simulink model "SA_50"  (R2021a)
settings: Solver=VariableStepAuto  StartTime=0.0  StopTime=simTime  RelTol=1e-3
model workspace (MAT data in the model file):
  SoC_0 = Simulink.Parameter
  SoC_0.DataType = 'auto'
  SoC_0.Dimensions = [0 0]
undefined symbols (not defined in the file or in its folder): Ion, Lithium, sigbuilder_block, slow_linearMPC
libraries: spsCurrentMeasurementLib x3, spsSeriesRLCBranchLib x2, spsDiodeLib x2, spspowerguiLib x1, spsBatteryLib x1, spsControlledCurrentSourceLib x1, spsFirstOrderFilterLib x1, spsFuelCellStackLib x1, spsMosfetLib x1, pid_lib x1, spsPWMGeneratorDCDCLib x1
settings Model: SimulationMode=accelerator  OrderedModelArguments=off  Creator=g  LastModifiedBy=leonardopalacios
settings SolverCC: ZeroCrossControl=DisableAll  ZeroCrossAlgorithm=Adaptive  AlgebraicLoopSolver=TrustRegion
settings DataIOCC: ReturnWorkspaceOutputs=off
settings DebuggingCC: SFMachineParentedDataDiag=warning  ArithmeticOperatorsInVariantConditions=warning
settings SFSimCC: SimUseLocalCustomCode=off  CustomCodeUndefinedFunction=UseInterfaceOnly
settings RTWCC: RTWUseLocalCustomCode=off
settings CodeAppCC: StateflowObjectComments=on
settings SimscapeCC: SimscapeNormalizeSystem=off

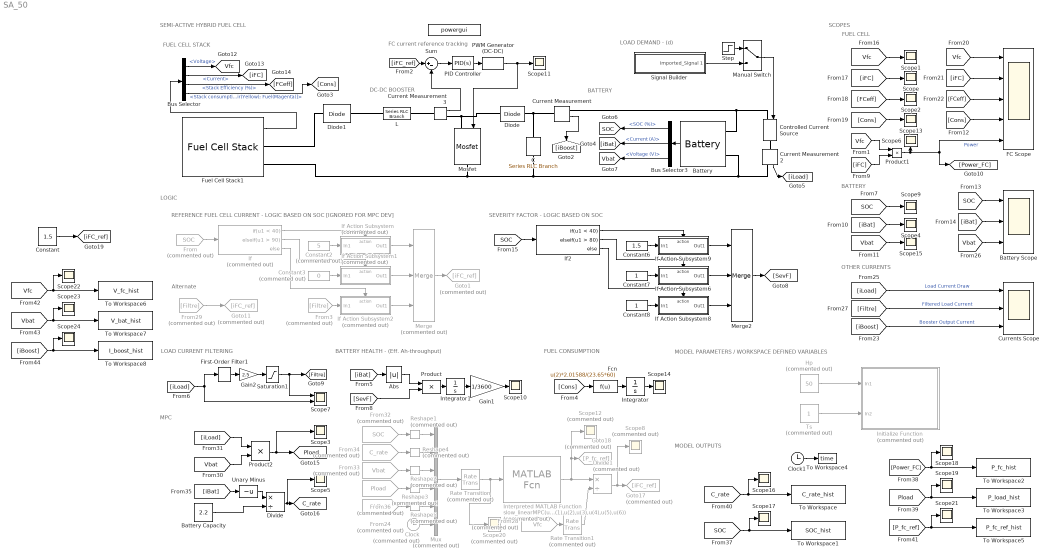
== system SA_50 ==
  note: MPC
  note: Alternate
  note: MODEL PARAMETERS / WORKSPACE DEFINED VARIABLES
  note: SCOPES
  note: SEMI-ACTIVE HYBRID FUEL CELL
  note: LOAD CURRENT FILTERING
  note: LOGIC
  note: LOAD DEMAND - (d)
  note: BATTERY
  note: REFERENCE FUEL CELL CURRENT - LOGIC BASED ON SOC [IGNORED FOR MPC DEV]
  note: FC current reference tracking
  note: DC-DC BOOSTER
  note: BATTERY
  note: FUEL CELL
  note: OTHER CURRENTS
  note: SEVERITY FACTOR - LOGIC BASED ON SOC
  note: FUEL CELL STACK
  note: BATTERY HEALTH - (Eff. Ah-throughput)
  note: FUEL CONSUMPTION
  note: MODEL OUTPUTS
  " " : spspowerguiLib/powergui  Priority=1  SimulationMode=Continuous  SampleTime=50e-6  frequency=60  Iterations=50  frequencyindice=0  Pbase=100e6  ErrMax=1e-4  UnitsV=kV  UnitsW=MW  buscounter=0  FunctionMessages=off  echomessages=off  EnableUseOfTLC=off  CurrentSourceSwitches=off  DisableSnubberDevices=off  DisableRonSwitches=off  DisableVfSwitches=off  DisplayEquations=off  AutomaticDiscreteSolvers=off  SolverType=Tustin/Backward Euler (TBE)  Interpol=off  ExternalGateDelay=off  methode=off  Ts=10  x0status=blocks  SPID=off  SwTol=0  HookPort=off  NonlinearTolerance=1e-4  nMaxIteration=100  ContinueOnMaxIteration=off  RestoreLinks=warning  ResistiveCurrentMeasurement=off  Frange=[0:2:500]  Ylog=off  Xlog=on  ShowGrid=off  save=off  variable=ZData  structure=0  ZoomFFT=off  StartTime=0.0  cycles=1  DisplayStyle=1  fundamental=60  FreqAxis=off  MaxFrequency=1000  frequencyindicesteady=1  RmsSteady=1  display=off
  Abs : Abs
  Battery : spsBatteryLib/Battery  BatType=Lithium-Ion  ShowTempParam=off  ThermalPreset=no  ShowAgeParam=off  NomV=40  NomQ=2.2  SOC=50  Batt_Tr=30  PresetModel=on  MaxQ=2.2  MinV=30  FullV=46.5595  Dis_rate=0.95652  R=0.18182  Normal_OP=1.9896  expZone="[43.2154     0.108087]"  current=[6.5 13 32.5]  Units=Time  Tci=20  NomT=25  T2=0  MaxQ2=2.208  FullV2=3.45  Normal_OP2=2.8  expZone2="[3.22        0.23]"  Rca=0.6  ti=1000  Dp=0  Neq0=0  Tsim=1e6  Ta1=25  Qeol=5.4*0.9  Reol=0.013333*1.2  Char_age=[2.3478, 3]  Dis_age=[2.3478, 10]  N1=1500  N2=10500  N3=1000  N4=1400  Ta2=45  N5=950
  Battery Capacity : Constant  Value=2.2
  "Battery Scope " : Scope  NumInputPorts=3
  Bus Selector : BusSelector  OutputSignals=Voltage,Current,Stack Efficiency (%),Stack consumption (Standard lpm) [Air(Yellow); Fuel(Magenta)]
  Bus Selector3 : BusSelector  OutputSignals=SOC (%),Current (A),Voltage (V)
  C : spsSeriesRLCBranchLib/Series RLC Branch  LConnTagsString=__new0  RConnTagsString=__new0  BranchType=C  Resistance=1  Inductance=100e-6  SetiL0=off  InitialCurrent=0  Capacitance=1000e-6  Setx0=off  InitialVoltage=0  Measurements=None
  Clock : Clock  Commented=on
  Clock1 : Clock
  Constant : Constant  Value=1.5
  Constant2 : Constant  Commented=on  Value=5
  Constant3 : Constant  Commented=on  Value=0
  Constant6 : Constant  Value=1.5
  Constant7 : Constant
  Constant8 : Constant
  Controlled Current Source : spsControlledCurrentSourceLib/Controlled Current Source  Initialize=off  Source_Type=DC  Amplitude=0  Phase=0  Frequency=0  Measurements=Current
  Current Measurement : spsCurrentMeasurementLib/Current Measurement  PhasorSimulation=off  OutputType=Complex  PSBequivalent=0
  Current Measurement2 : spsCurrentMeasurementLib/Current Measurement  PhasorSimulation=off  OutputType=Complex  PSBequivalent=0
  Current Measurement3 : spsCurrentMeasurementLib/Current Measurement  PhasorSimulation=off  OutputType=Complex  PSBequivalent=0
  "Currents Scope " : Scope  NumInputPorts=3
  Diode : spsDiodeLib/Diode  Ron=0.001  Lon=0  Vf=0.8  IC=0  UseSnubber=off  Rs=500  Cs=250e-9  Measurements=off
  Diode1 : spsDiodeLib/Diode  Ron=0.001  Lon=0  Vf=0.8  IC=0  UseSnubber=off  Rs=500  Cs=250e-9  Measurements=off
  Divide : Product  Inputs=*/
  Divide1 : Product  Commented=on  Inputs=*/
  FC Scope : Scope  NumInputPorts=5
  Fcn : Fcn  Expr=u(2)*2.01588/(23.65*60)
  First-Order Filter1 : spsFirstOrderFilterLib/First-Order Filter  FilterType=Lowpass  Tc=5  Ts=0  Initialize=on  Vac_Init=[0, 0, 60]  Vdc_Init=1.1  PlotResponse=off  FreqRange="[0,  200,  1]"
  From : From  Commented=on  GotoTag=SOC
  From24 : From  Commented=on  GotoTag=Vfc  TagVisibility=global
  From28 : From  Commented=on  GotoTag=Vfc  TagVisibility=global
  From29 : From  Commented=on  GotoTag=Filtre
  From3 : From  Commented=on  GotoTag=Filtre
  From32 : From  Commented=on  GotoTag=SOC  TagVisibility=global
  From33 : From  Commented=on  GotoTag=Vbat  TagVisibility=global
  From34 : From  Commented=on  GotoTag=C_rate  TagVisibility=global
  From36 : From  Commented=on  GotoTag=Pload  TagVisibility=global
  Fuel Cell Stack1 : spsFuelCellStackLib/Fuel Cell Stack  PresetModel=No (User-Defined)  FcType=0  Detailed=Detailed  Eoc="[18  15]"  NomVI="[4        12.5]"  EndVI="[5   12]"  Nc=20  n=46  TOp=25  AirFr=20  SuppPress="[0.35           0.3]"  Comp="[99.95           21            1]"  SignX=off  SignY=off  FlowRateH2=off  FlowRateAir=off  SystemTemp=off  SystemPH2=off  SystemPAir=off  FCDyn=off  FC_tau=1  Peak_O2=80  V_Under=10
      settings: SourceProductBaseCode=PS
  Gain1 : Gain  Gain=1/3600
  Gain2 : Gain  Gain=2.5
  Goto1 : Goto  Commented=on  GotoTag=iFC_ref
  Goto11 : Goto  Commented=on  GotoTag=iFC_ref
  Goto17 : Goto  Commented=on  GotoTag=iFC_ref
  Goto18 : Goto  Commented=on  GotoTag=P_fc_ref
  Hp : Constant  Commented=on  Value=50
  If : If  Commented=on  IfExpression=u1 < 40  ElseIfExpressions=u1 > 90
  If Action Subsystem : Subsystem  Commented=on  TreatAsAtomicUnit=on
  If Action Subsystem1 : Subsystem  Commented=on  TreatAsAtomicUnit=on
  If Action Subsystem2 : Subsystem  Commented=on  TreatAsAtomicUnit=on
  If Action Subsystem6 : Subsystem  TreatAsAtomicUnit=on
  If Action Subsystem8 : Subsystem  TreatAsAtomicUnit=on
  If Action Subsystem9 : Subsystem  TreatAsAtomicUnit=on
  If2 : If  IfExpression=u1 < 40  ElseIfExpressions=u1 > 80
  Initialize Function : Subsystem  Commented=on  TreatAsAtomicUnit=on
  Integrator : Integrator
  Integrator1 : Integrator
  Interpreted MATLAB Function : MATLABFcn  Commented=on  MATLABFcn=slow_linearMPC(u(1),u(2),u(3),u(4),u(5),u(6))
  L : spsSeriesRLCBranchLib/Series RLC Branch  LConnTagsString=__new0  RConnTagsString=__new0  BranchType=L  Resistance=1  Inductance=100e-3  SetiL0=off  InitialCurrent=0  Capacitance=1e-6  Setx0=off  InitialVoltage=0  Measurements=None
  Manual Switch : ManualSwitch
  Merge : Merge  Commented=on  Inputs=3
  Merge2 : Merge  Inputs=3
  Mosfet : spsMosfetLib/Mosfet  Ron=0.1  Lon=0  Rd=0.01  Vfd=0  IC=0  Rs=1e5  Cs=inf  Measurements=off
  Mux : Mux  Commented=on  Inputs=6
  PID Controller : pid_lib/PID Controller  Controller=PID  Form=Parallel  TimeDomain=Continuous-time  UseExternalTs=off  SampleTime=-1  IntegratorMethod=Forward Euler  FilterMethod=Forward Euler  ControllerParametersSource=internal  P=1  I=2  D=0  UseFilter=on  N=100  TunerSelectOption=Transfer Function Based (PID Tuner App)  InitialConditionSource=internal  InitialConditionForIntegrator=0  InitialConditionForFilter=0  DifferentiatorICPrevScaledInput=0  ExternalReset=none  TrackingMode=off  Kt=1  LimitOutput=off  SatLimitsSource=internal  UpperSaturationLimit=inf  LowerSaturationLimit=-inf  LinearizeAsGain=on  AntiWindupMode=none  Kb=1  POutMin=[]  POutMax=[]  IOutMin=[]  IOutMax=[]  DOutMin=[]  DOutMax=[]  NOutMin=[]  NOutMax=[]  SumOutMin=[]  SumOutMax=[]  SaturationOutMin=[]  SaturationOutMax=[]  PParamMin=[]  PParamMax=[]  IParamMin=[]  IParamMax=[]  DParamMin=[]  DParamMax=[]  NParamMin=[]  NParamMax=[]  KbParamMin=[]  KbParamMax=[]  KtParamMin=[]  KtParamMax=[]  KbOutMin=[]  KbOutMax=[]  KtOutMin=[]  KtOutMax=[]  IntegratorOutMin=[]  IntegratorOutMax=[]  FilterOutMin=[]  FilterOutMax=[]  SumI1OutMin=[]  SumI1OutMax=[]  SumI2OutMin=[]  SumI2OutMax=[]  SumI3OutMin=[]  SumI3OutMax=[]  SumI4OutMin=[]  SumI4OutMax=[]  SumDOutMin=[]  SumDOutMax=[]  DifferentiatorOutMin=[]  DifferentiatorOutMax=[]  FilterDiffOutCoefMin=[]  FilterDiffOutCoefMax=[]  ReciprocalOutMin=[]  ReciprocalOutMax=[]  SumDenOutMin=[]  SumDenOutMax=[]  SumNumOutMin=[]  SumNumOutMax=[]  DivideOutMin=[]  DivideOutMax=[]  UdiffTsProdOutMin=[]  UdiffTsProdOutMax=[]  NTsProdOutMin=[]  NTsProdOutMax=[]  UintegralTsProdOutMin=[]  UintegralTsProdOutMax=[]  UngainTsProdOutMin=[]  UngainTsProdOutMax=[]  IntegratorContinuousStateAttributes=''  IntegratorStateMustResolveToSignalObject=off  IntegratorRTWStateStorageClass=Auto  FilterContinuousStateAttributes=''  FilterStateMustResolveToSignalObject=off  FilterRTWStateStorageClass=Auto  ParallelPVariant=InternalParameters  IdealPVariant=Disabled  IVariant=InternalParameters  DVariant=InternalParameters  IntegratorVariant=Continuous  SatVariant=Disabled  AWVariant=Passthrough  PCopyVariant=Disabled  TRVariant=Disabled  FdbkBlocksVariant=Forward  IdealPFdbkVariant=Disabled  SatFdbkVariant=Disabled  DerivativeFilterVariant=ContFilter  NVariant=InternalParameters  NCopyVariant=Disabled  FilterICVariant=InternalICsFilter  IntegratorICVariant=InternalICs  ExternalResetVariant=Disabled  TRSumVariant=Passthrough  SumFdbkVariant=Disabled  SumVariant=Sum_PID  TsampFilterVariant=InternalTs  TsampNgainVariant=Passthrough  TsampIntegralVariant=Passthrough  ExternalSaturationOutDataTypeStr=Inherit: Same as second input
  PWM Generator (DC-DC) : spsPWMGeneratorDCDCLib/PWM Generator (DC-DC)  Fsw=1000  Ts=0
  Product : Product
  Product1 : Product
  Product2 : Product
  Rate Transition : RateTransition  Commented=on  OutPortSampleTime=Ts
  Rate Transition1 : RateTransition  Commented=on  OutPortSampleTime=Ts
  Reshape{1..5} (5 alike) : Reshape  Commented=on  OutputDimensionality=Customize  OutputDimensions=1
  Saturation1 : Saturate  UpperLimit=5  LowerLimit=0
  Scope{,1..6,9..11,13..19,21..24} (21 alike) : Scope
  Scope12 : Scope  Commented=on
  Scope20 : Scope  Commented=on
  Scope7 : Scope  NumInputPorts=2
  Scope8 : Scope  Commented=on
  Signal Builder : Subsystem  Tag=STV Subsys  LoadFcn=sigbuilder_block('load');  StartFcn=sigbuilder_block('start');  StopFcn=sigbuilder_block('stop');  ClipboardFcn=sigbuilder_block('clipboard');  mask(Sigbuilder block){tuvar=[0:10]}
      mask help: Simulink:masks:SigbuilderBlock_MD
      mask init:
      | if ~strcmp(get_param(bdroot(gcbh),'SimulationStatus'),'stopped') tuvar = sigbuilder_block('maskInit'); end
      settings: CopyFcn=sigbuilder_block('copy');  DeleteFcn=sigbuilder_block('delete');  ModelCloseFcn=sigbuilder_block('modelClose');  PreSaveFcn=sigbuilder_block('preSave');  PauseFcn=sigbuilder_block('pause');  ContinueFcn=sigbuilder_block('continue');  NameChangeFcn=sigbuilder_block('namechange');  OpenFcn=sigbuilder_block('open',[214 20 1706 550 ]);  CloseFcn=sigbuilder_block('close');
      mask Display: plot(0, 0, 100, 100,[2, 2, 32, 32, 2], [68, 8, 8, 68, 68],[32, 2], [38, 38], [32, 19, 2],[53, 60, 44], [32, 17, 17, 2],[16, 16, 31, 31]);txt = getActiveGroup(gcbh);text(2, 100, txt,'verticalAlignment', 'top');
  Step : Step  Time=0  After=0.6  SampleTime=0
  Sum : Sum  Inputs=|+-
  To Workspace : ToWorkspace  VariableName=C_rate_hist  SaveFormat=Timeseries  SampleTime=-1
  To Workspace1 : ToWorkspace  VariableName=SOC_hist  SaveFormat=Timeseries  SampleTime=-1
  To Workspace2 : ToWorkspace  VariableName=P_fc_hist  SaveFormat=Timeseries  SampleTime=-1
  To Workspace3 : ToWorkspace  VariableName=P_load_hist  SaveFormat=Timeseries  SampleTime=-1
  To Workspace4 : ToWorkspace  VariableName=time  SaveFormat=Timeseries  SampleTime=-1
  To Workspace5 : ToWorkspace  VariableName=P_fc_ref_hist  SaveFormat=Timeseries  SampleTime=-1
  To Workspace6 : ToWorkspace  VariableName=V_fc_hist  SaveFormat=Timeseries  SampleTime=-1
  To Workspace7 : ToWorkspace  VariableName=V_bat_hist  SaveFormat=Timeseries  SampleTime=-1
  To Workspace8 : ToWorkspace  VariableName=I_boost_hist  SaveFormat=Timeseries  SampleTime=-1
  Ts : Constant  Commented=on
  Unary Minus : UnaryMinus
  tag scope: C_rate=global, Pload=global, SOC=global, Vbat=global, Vfc=global
  wires:
  Fuel Cell Stack1/1 -> Bus Selector/1
  [iFC_ref] -> Sum/1
  PWM Generator (DC-DC)/1 -> Mosfet/1, Scope11/1
  Current Measurement3/1 -> Sum/2
  From/1 -> If/1
  If/1 -> If Action Subsystem/Action
  If/2 -> If Action Subsystem1/Action
  If/3 -> If Action Subsystem2/Action
  Constant2/1 -> If Action Subsystem/1(In1)
  Constant3/1 -> If Action Subsystem1/1(In1)
  From3/1 -> If Action Subsystem2/1(In1)
  If Action Subsystem/1(Out1) -> Merge/1
  If Action Subsystem1/1(Out1) -> Merge/2
  If Action Subsystem2/1(Out1) -> Merge/3
  Merge/1 -> Goto1/1
  [Cons] -> Fcn/1
  Fcn/1 -> Integrator/1
  Integrator/1 -> Scope14/1
  [iBat] -> Abs/1
  Abs/1 -> Product/1
  [SevF] -> Product/2
  Product/1 -> Integrator1/1
  Bus Selector/4 -> [Cons]  "<Stack consumption (Standard lpm) [Air(Yellow); Fuel(Magenta)]>"
  Bus Selector/1 -> [Vfc]  "<Voltage>"
  Bus Selector/2 -> [iFC]  "<Current>"
  Bus Selector/3 -> [FCeff]  "<Stack Efficiency (%)>"
  [SOC] -> Scope9/1
  [iBat] -> Scope4/1
  [Vbat] -> Scope15/1
  [Vfc] -> Scope1/1
  [iFC] -> Scope/1
  [FCeff] -> Scope2/1
  [Cons] -> Scope13/1
  [Vfc] -> FC Scope/1
  [iFC] -> FC Scope/2
  [FCeff] -> FC Scope/3
  [Cons] -> FC Scope/4
  [SOC] -> "Battery Scope "/1
  [Vbat] -> "Battery Scope "/3
  Sum/1 -> PID Controller/1
  PID Controller/1 -> PWM Generator (DC-DC)/1
  Integrator1/1 -> Gain1/1
  Gain1/1 -> Scope10/1
  [Vfc] -> Product1/1
  [iFC] -> Product1/2
  [iBat] -> "Battery Scope "/2
  Product1/1 -> FC Scope/5, [Power_FC], Scope6/1  "Power"
  If2/3 -> If Action Subsystem8/Action
  If2/1 -> If Action Subsystem9/Action
  Constant6/1 -> If Action Subsystem9/1(In1)
  Merge2/1 -> [SevF]
  Constant8/1 -> If Action Subsystem8/1(In1)
  If Action Subsystem9/1(Out1) -> Merge2/1
  Constant7/1 -> If Action Subsystem6/1(In1)
  If Action Subsystem6/1(Out1) -> Merge2/2
  [SOC] -> If2/1
  If2/2 -> If Action Subsystem6/Action
  If Action Subsystem8/1(Out1) -> Merge2/3
  Gain2/1 -> Saturation1/1
  Saturation1/1 -> [Filtre], Scope7/1
  First-Order Filter1/1 -> Gain2/1
  [iLoad] -> Scope7/2, First-Order Filter1/1
  Current Measurement2/1 -> [iLoad]
  Current Measurement/1 -> [iBoost]
  [iLoad] -> "Currents Scope "/1  "Load Current Draw"
  [Filtre] -> "Currents Scope "/2  "Filtered Load Current"
  [iBoost] -> "Currents Scope "/3  "Booster Output Current"
  From29/1 -> Goto11/1
  Step/1 -> Manual Switch/1
  Signal Builder/1(Imported_Signal 1) -> Manual Switch/2
  Manual Switch/1 -> Controlled Current Source/1
  [Vbat] -> Product2/2
  [iLoad] -> Product2/1
  Product2/1 -> Scope3/1, [Pload]
  Battery Capacity/1 -> Divide/2
  Divide/1 -> Scope5/1, [C_rate]
  Mux/1 -> Rate Transition/1
  Divide1/1 -> Scope8/1, Goto17/1
  Battery/1 -> Bus Selector3/1
  Bus Selector3/1 -> [SOC]  "<SOC (%)>"
  Bus Selector3/2 -> [iBat]  "<Current (A)>"
  Bus Selector3/3 -> [Vbat]  "<Voltage (V)>"
  Rate Transition/1 -> Scope20/1, Interpreted MATLAB Function/1
  From32/1 -> Reshape1/1
  Reshape1/1 -> Mux/1
  From33/1 -> Reshape2/1
  Reshape2/1 -> Mux/3
  From36/1 -> Reshape3/1
  Reshape3/1 -> Mux/4
  From34/1 -> Reshape4/1
  Reshape4/1 -> Mux/2
  Clock/1 -> Mux/6
  From24/1 -> Reshape5/1
  Reshape5/1 -> Mux/5
  Interpreted MATLAB Function/1 -> Goto18/1, Scope12/1, Divide1/1
  [iBat] -> Unary Minus/1
  Unary Minus/1 -> Divide/1
  From28/1 -> Rate Transition1/1
  Rate Transition1/1 -> Divide1/2
  [C_rate] -> To Workspace/1, Scope16/1
  [SOC] -> Scope17/1, To Workspace1/1
  [Power_FC] -> To Workspace2/1, Scope18/1
  [Pload] -> Scope19/1, To Workspace3/1
  Hp/1 -> Initialize Function/1(In1)
  Ts/1 -> Initialize Function/2(In2)
  Clock1/1 -> To Workspace4/1
  [P_fc_ref] -> Scope21/1, To Workspace5/1
  Constant/1 -> [iFC_ref]
  [Vbat] -> Scope23/1, To Workspace7/1
  [Vfc] -> To Workspace6/1, Scope22/1
  [iBoost] -> Scope24/1, To Workspace8/1
  connections:
  Diode/LConn1 -- Current Measurement3/RConn1 -- Mosfet/LConn1
  C/LConn1 -- Current Measurement/LConn1 -- Diode/RConn1
  Current Measurement2/RConn1 -- Battery/LConn2 -- C/RConn1 -- Fuel Cell Stack1/RConn2 -- Mosfet/RConn1
  Current Measurement/RConn1 -- Battery/LConn1 -- Controlled Current Source/LConn1
  Controlled Current Source/RConn1 -- Current Measurement2/LConn1
  L/RConn1 -- Current Measurement3/LConn1
  Fuel Cell Stack1/RConn1 -- Diode1/LConn1
  Diode1/RConn1 -- L/LConn1

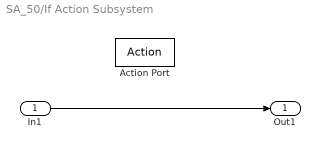
== system SA_50/If Action Subsystem ==
  In1 : Inport
  Action Port : ActionPort  ActionPortLabel=if(u1 < 40)
  Out1 : Outport
  wires:
  In1/1 -> Out1/1

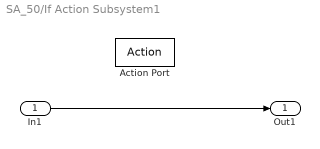
== system SA_50/If Action Subsystem1 ==
  In1 : Inport
  Action Port : ActionPort  ActionPortLabel=elseif(u1 > 90)
  Out1 : Outport
  wires:
  In1/1 -> Out1/1

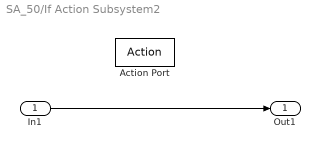
== system SA_50/If Action Subsystem2 ==
  In1 : Inport
  Action Port : ActionPort  ActionPortLabel=else
  Out1 : Outport
  wires:
  In1/1 -> Out1/1

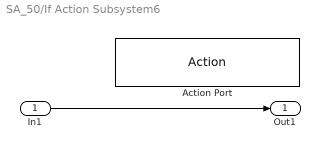
== system SA_50/If Action Subsystem6 ==
  In1 : Inport
  Action Port : ActionPort  ActionPortLabel=elseif(u1 > 80)
  Out1 : Outport
  wires:
  In1/1 -> Out1/1

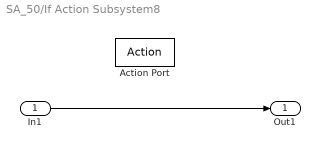
== system SA_50/If Action Subsystem8 ==
  In1 : Inport
  Action Port : ActionPort  ActionPortLabel=else
  Out1 : Outport
  wires:
  In1/1 -> Out1/1

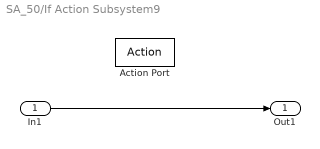
== system SA_50/If Action Subsystem9 ==
  In1 : Inport
  Action Port : ActionPort  ActionPortLabel=if(u1 < 40)
  Out1 : Outport
  wires:
  In1/1 -> Out1/1

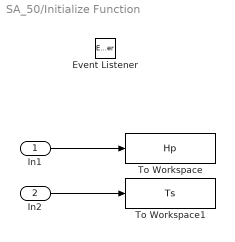
== system SA_50/Initialize Function ==
  In1 : Inport
  In2 : Inport  Port=2
  Event Listener : EventListener  DisableCoverage=on  EventName=reset
  To Workspace : ToWorkspace  VariableName=Hp  SaveFormat=Timeseries  SampleTime=-1
  To Workspace1 : ToWorkspace  VariableName=Ts  SaveFormat=Timeseries  SampleTime=-1
  wires:
  In2/1 -> To Workspace1/1
  In1/1 -> To Workspace/1

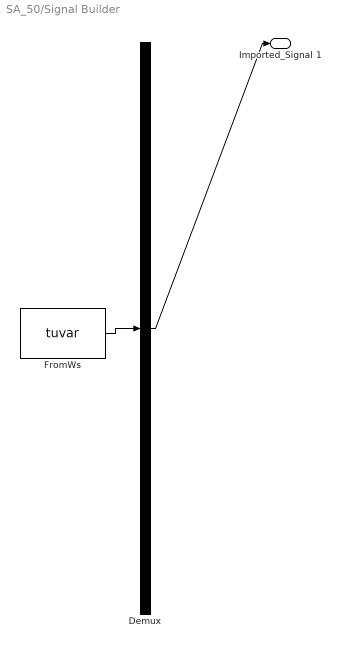
== system SA_50/Signal Builder ==
  Demux : Demux  Tag=STV Demux  Outputs=1
      settings: DisplayOption=none
  FromWs : FromWorkspace  Tag=STV FromWs  VariableName=tuvar
      SigBuilderData=|
      | common.afterFinalStr = 'Extrapolate'
      | common.sampleTime = 0
      | dataSet.timeRange = [0 1498.3]
      | dataSet.name = 'Combi12'
      | sbobj.Name = 'Signal Builder'
      | sbobj.Groups.Name = 'Combi12'
      | sbobj.Groups.Signals.Name = 'Imported_Signal 1'
      | sbobj.Groups.Signals.XData = [0 0.1 0.2 0.3 0.4 0.5 0.6 0.7 0.8 0.9 1 1.1 ... (14984 elements, 1x14984)]
      | sbobj.Groups.Signals.YData = [1.0569 1.1309 1.171 1.162 0.9589 1.143 1.056 1.261 1.1779 1.1458 1.2318 1.238 ... (14984 elements, 1x14984)]
      | sbobj.Groups.TimeRange = [0 1498.3]
  Imported_Signal 1 : Outport  Tag=STV Outport
  wires:
  FromWs/1 -> Demux/1
  Demux/1 -> Imported_Signal 1/1
